simulink model "PPRZ2l"  (R2024b)
settings: Solver=VariableStepAuto  StartTime=0.0  StopTime=10.0  RelTol=1e-3
settings Model: Creator=kkajak  LastModifiedBy=feder
settings SolverCC: AlgebraicLoopSolver=TrustRegion
settings DataIOCC: ReturnWorkspaceOutputs=off
settings DebuggingCC: UnconnectedInputMsg=warning  UnconnectedOutputMsg=warning  UnconnectedLineMsg=warning  ArithmeticOperatorsInVariantConditions=warning
settings ModelReferenceCC: EnableRefExpFcnMdlSchedulingChecks=on
settings SFSimCC: SimUseLocalCustomCode=off  CustomCodeUndefinedFunction=UseInterfaceOnly
settings RTWCC: RTWUseLocalCustomCode=off  GPUComputeCapability=3.5
settings CodeAppCC: StateflowObjectComments=on

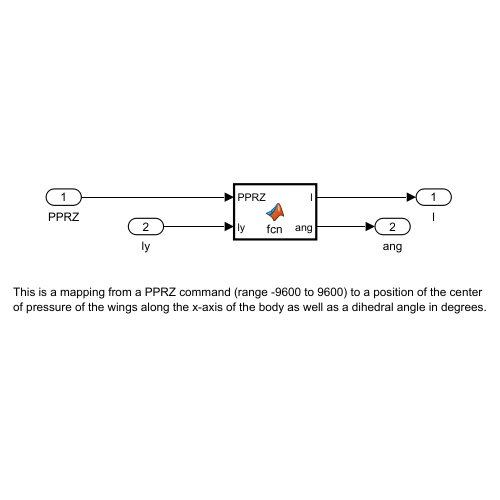
[thumbnail: Simulink's stored preview of the top-level diagram]
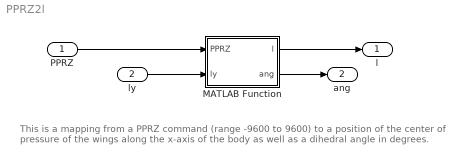
== system PPRZ2l ==
  note: This is a mapping from a PPRZ command (range -9600 to 9600) to a position of the center
      | of pressure of the wings along the x-axis of the body as well as a dihedral angle in degrees.
  PPRZ : Inport
  "ly " : Inport  Port=2
  MATLAB Function : MATLAB Function  TreatAsAtomicUnit=on
  l : Outport
  ang : Outport  Port=2
  wires:
  PPRZ/1 -> MATLAB Function/1(PPRZ)
  "ly "/1 -> MATLAB Function/2(ly)
  MATLAB Function/1(l) -> l/1
  MATLAB Function/2(ang) -> ang/1

== matlab function PPRZ2l/MATLAB Function ==
  data: PPRZ input; l output; ly input; ang output
function [l,ang] = fcn(PPRZ,ly)

ang = -PPRZ/100*18;
l = ly*sind(ang);
